simulink model "dc_servo_speed_estimation"  (R2020b)
settings: Solver=ode5  StartTime=0.0  StopTime=.25  FixedStep=.00001  RelTol=1e-6  AbsTol=1e-6
values from neighbouring files (symbols this model uses):
  encoder = 2000    [dc_servo_HighGainCommand_data.m]    (also in dc_servo_speed_estimation_data.m)
  f = 4e-4    (= 0.0004)    [dc_servo_HighGainCommand_data.m]    (also in dc_servo_speed_estimation_data.m)
  imax = 5    [dc_servo_HighGainCommand_data.m]    (also in dc_servo_speed_estimation_data.m)
  integrator_saturation = 10000    [dc_servo_HighGainCommand_data.m]    (also in dc_servo_speed_estimation_data.m)
  J = 6.0e-5    (= 6e-05)    [dc_servo_HighGainCommand_data.m]    (also in dc_servo_speed_estimation_data.m)
  KI = k*k    (= 10000)    [dc_servo_HighGainCommand_data.m]    (also in dc_servo_speed_estimation_data.m)
  Kp = k    (= 100)    [dc_servo_HighGainCommand_data.m]    (also in dc_servo_speed_estimation_data.m = 200)
  KT = 0.07    [dc_servo_HighGainCommand_data.m]    (also in dc_servo_speed_estimation_data.m)
  L = 0.002    [dc_servo_HighGainCommand_data.m]    (also in dc_servo_speed_estimation_data.m)
  l1 = p1 + p2 + p3 - f/J    (= 893.333333333)    [dc_servo_speed_estimation_data.m]
  l2 = p1*p2 + p1*p3 + p2*p3 -l1*(f/J)    (= 264044.444444)    [dc_servo_speed_estimation_data.m]
  l3 = -p1*p2*p3    (= -27000000)    [dc_servo_speed_estimation_data.m]
  load_torque = 0    [dc_servo_HighGainCommand_data.m]    (also in dc_servo_speed_estimation_data.m)
  omega0 = 0    [dc_servo_HighGainCommand_data.m]    (also in dc_servo_speed_estimation_data.m)
  R = 2    [dc_servo_HighGainCommand_data.m]    (also in dc_servo_speed_estimation_data.m)
  theta0 = 0    [dc_servo_HighGainCommand_data.m]    (also in dc_servo_speed_estimation_data.m)
  Ts = 0.001    [dc_servo_HighGainCommand_data.m]    (also in dc_servo_speed_estimation_data.m)
  vmax = 40    [dc_servo_HighGainCommand_data.m]    (also in dc_servo_speed_estimation_data.m)
libraries: simulink x1
settings Model: ExtModeTrigMode=oneshot  ExtModeArmWhenConnect=off  Creator=johnchiasson  LastModifiedBy=johnchiasson
settings DataIOCC: SaveFormat=Array  SignalLoggingSaveFormat=ModelDataLogs  SaveOutput=off  SaveTime=off  ReturnWorkspaceOutputs=off  SignalLoggingName=sigsOut
settings OptimizationCC: BlockReduction=off  BooleanDataType=off
settings DebuggingCC: SaveWithParameterizedLinksMsg=none  UnderspecifiedInitializationDetection=Classic  MergeDetectMultiDrivingBlocksExec=none  SignalResolutionControl=TryResolveAllWithWarning  MultiTaskDSMMsg=warning  MultiTaskCondExecSysMsg=none
settings HardwareCC: ProdBitPerPointer=32  ProdBitPerSizeT=32  ProdBitPerPtrDiffT=32  ProdLargestAtomicFloat=None  ProdIntDivRoundTo=Undefined  ProdEndianess=Unspecified  ProdWordSize=32  ProdHWDeviceType=32-bit Generic  TargetUnknown=on
settings ModelReferenceCC: PropagateSignalLabelsOutOfModel=off
settings GRTTargetCC: CombineOutputUpdateFcns=off  GRTInterface=on
settings ConfigComp: CovMetricSettings=dw  CovSaveCumulativeToWorkspaceVar=on  CovSaveSingleToWorkspaceVar=on

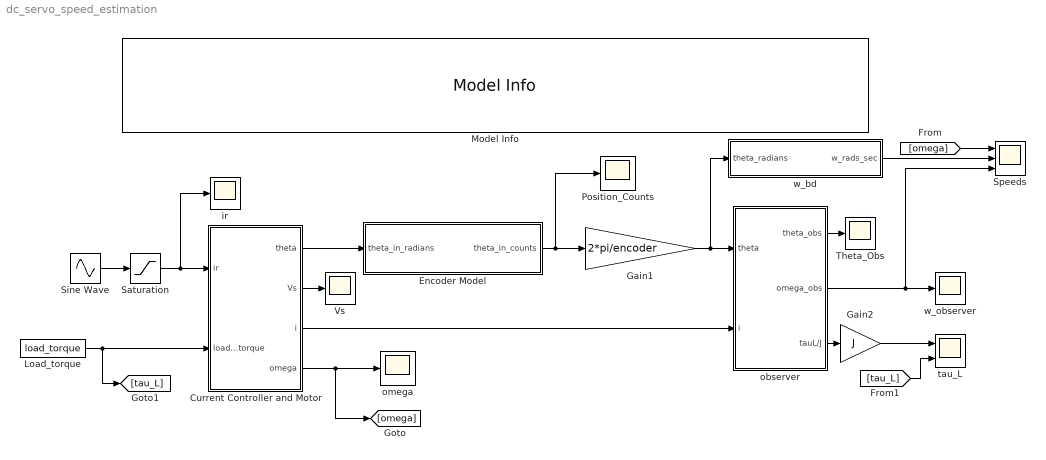
== system dc_servo_speed_estimation ==
  Current Controller and Motor : Subsystem
  Encoder Model : Subsystem
  Gain1 : Gain  Gain=2*pi/encoder  SaturateOnIntegerOverflow=on  OutDataTypeStr=Inherit: Same as input  ParamDataTypeStr=Inherit: Same as input
  Gain2 : Gain  Gain=J  SaturateOnIntegerOverflow=on  OutDataTypeStr=Inherit: Same as input  ParamDataTypeStr=Inherit: Same as input
  Load_torque : Constant  Value=load_torque
  Model Info : simulink/Model-Wide Utilities/Model Info  Frame=on  DisplayStringWithTags=|  HorizontalTextAlignment=Center  LeftAlignmentValue=0.5
      | Backward Difference Speed Estimator
      |  and 
      | Speed & Load Torque Estimator
  Position_Counts : Scope
  Saturation : Saturate  UpperLimit=imax  LowerLimit=-imax
  Sine Wave : Sin  Amplitude=0.5  Frequency=2*pi/0.2  SampleTime=0
  Speeds : Scope  NumInputPorts=3
  Theta_Obs : Scope
  Vs : Scope
  ir : Scope
  observer : Subsystem
  omega : Scope
  tau_L : Scope  NumInputPorts=2
  w_bd : Subsystem
  w_observer : Scope
  wires:
  Current Controller and Motor/4(omega) -> [omega], omega/1
  Load_torque/1 -> [tau_L], Current Controller and Motor/2(load_torque)
  Current Controller and Motor/2(Vs) -> Vs/1
  Current Controller and Motor/1(theta) -> Encoder Model/1(theta_in_radians)
  Saturation/1 -> Current Controller and Motor/1(ir), ir/1
  Gain1/1 -> w_bd/1(theta_radians), observer/1(theta)
  Encoder Model/1(theta_in_counts) -> Gain1/1, Position_Counts/1
  observer/1(theta_obs) -> Theta_Obs/1
  Current Controller and Motor/3(i) -> observer/2(i)
  observer/2(omega_obs) -> Speeds/3, w_observer/1
  w_bd/1(w_rads_sec) -> Speeds/2
  Sine Wave/1 -> Saturation/1
  observer/3(tauL/J) -> Gain2/1
  Gain2/1 -> tau_L/1
  [omega] -> Speeds/1
  [tau_L] -> tau_L/2

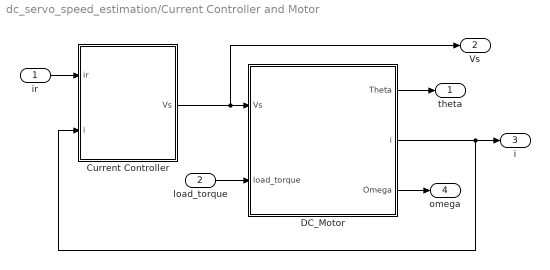
== system dc_servo_speed_estimation/Current Controller and Motor ==
  ir : Inport
  load_torque : Inport  Port=2
  Current Controller : Subsystem
  DC_Motor : Subsystem
  theta : Outport
  Vs : Outport  Port=2
  i : Outport  Port=3
  omega : Outport  Port=4
  wires:
  Current Controller/1(Vs) -> DC_Motor/1(Vs), Vs/1
  ir/1 -> Current Controller/1(ir)
  DC_Motor/3(Omega) -> omega/1
  DC_Motor/1(Theta) -> theta/1
  DC_Motor/2(i) -> i/1, Current Controller/2(i)
  load_torque/1 -> DC_Motor/2(load_torque)

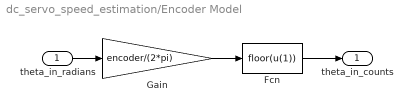
== system dc_servo_speed_estimation/Encoder Model ==
  theta_in_radians : Inport
  Fcn : Fcn  Expr=floor(u(1))
  Gain : Gain  Gain=encoder/(2*pi)  SaturateOnIntegerOverflow=on  OutDataTypeStr=Inherit: Same as input  ParamDataTypeStr=Inherit: Same as input
  theta_in_counts : Outport
  wires:
  Gain/1 -> Fcn/1
  theta_in_radians/1 -> Gain/1
  Fcn/1 -> theta_in_counts/1

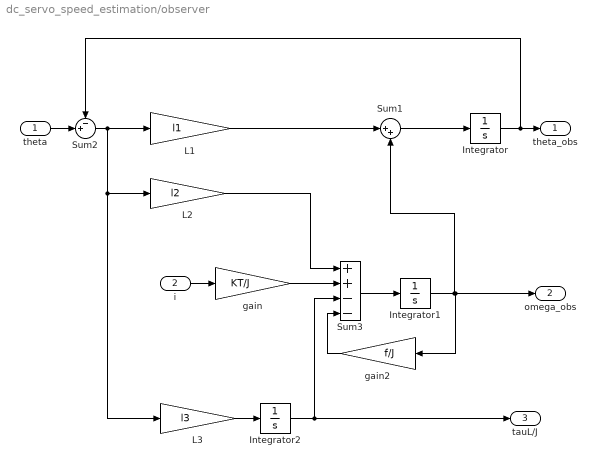
== system dc_servo_speed_estimation/observer ==
  theta : Inport
  i : Inport  Port=2
  Integrator : Integrator
  Integrator1 : Integrator
  Integrator2 : Integrator
  L1 : Gain  Gain=l1  SaturateOnIntegerOverflow=on  OutDataTypeStr=Inherit: Same as input  ParamDataTypeStr=Inherit: Same as input
  L2 : Gain  Gain=l2  SaturateOnIntegerOverflow=on  OutDataTypeStr=Inherit: Same as input  ParamDataTypeStr=Inherit: Same as input
  "L3 " : Gain  Gain=l3  SaturateOnIntegerOverflow=on  OutDataTypeStr=Inherit: Same as input  ParamDataTypeStr=Inherit: Same as input
  Sum1 : Sum  Inputs=|++  InputSameDT=on  SaturateOnIntegerOverflow=on  OutDataTypeStr=Inherit: Same as first input
  Sum2 : Sum  Inputs=-+|  InputSameDT=on  SaturateOnIntegerOverflow=on  OutDataTypeStr=Inherit: Same as first input
  Sum3 : Sum  Inputs=++--  InputSameDT=on  SaturateOnIntegerOverflow=on  OutDataTypeStr=Inherit: Same as first input
  gain : Gain  Gain=KT/J  SaturateOnIntegerOverflow=on  OutDataTypeStr=Inherit: Same as input  ParamDataTypeStr=Inherit: Same as input
  gain2 : Gain  Gain=f/J  SaturateOnIntegerOverflow=on  OutDataTypeStr=Inherit: Same as input  ParamDataTypeStr=Inherit: Same as input
  theta_obs : Outport
  omega_obs : Outport  Port=2
  tauL/J : Outport  Port=3
  wires:
  Sum2/1 -> L1/1, "L3 "/1, L2/1
  Sum3/1 -> Integrator1/1
  Integrator1/1 -> omega_obs/1, gain2/1, Sum1/2
  L1/1 -> Sum1/1
  Sum1/1 -> Integrator/1
  Integrator/1 -> Sum2/1, theta_obs/1
  theta/1 -> Sum2/2
  L2/1 -> Sum3/1
  gain/1 -> Sum3/2
  i/1 -> gain/1
  "L3 "/1 -> Integrator2/1
  Integrator2/1 -> Sum3/3, tauL/J/1
  gain2/1 -> Sum3/4

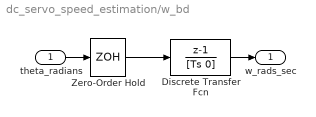
== system dc_servo_speed_estimation/w_bd ==
  theta_radians : Inport
  Discrete Transfer Fcn : DiscreteTransferFcn  Numerator=[1 -1]  Denominator=[Ts 0]  SampleTime=Ts
  Zero-Order Hold : ZeroOrderHold  SampleTime=Ts
  w_rads_sec : Outport
  wires:
  Discrete Transfer Fcn/1 -> w_rads_sec/1
  Zero-Order Hold/1 -> Discrete Transfer Fcn/1
  theta_radians/1 -> Zero-Order Hold/1

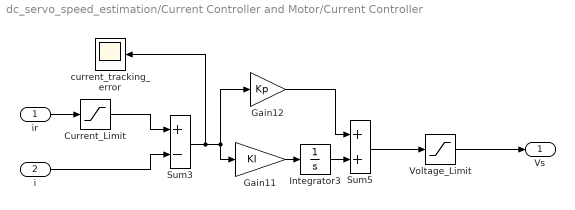
== system dc_servo_speed_estimation/Current Controller and Motor/Current Controller ==
  ir : Inport
  i : Inport  Port=2
  Current_Limit : Saturate  UpperLimit=imax  LowerLimit=-imax
  Gain11 : Gain  Gain=KI  SaturateOnIntegerOverflow=on  OutDataTypeStr=Inherit: Same as input  ParamDataTypeStr=Inherit: Same as input
  Gain12 : Gain  Gain=Kp  SaturateOnIntegerOverflow=on  OutDataTypeStr=Inherit: Same as input  ParamDataTypeStr=Inherit: Same as input
  Integrator3 : Integrator
  Sum3 : Sum  Inputs=+-  InputSameDT=on  SaturateOnIntegerOverflow=on  OutDataTypeStr=Inherit: Same as first input
  Sum5 : Sum  InputSameDT=on  SaturateOnIntegerOverflow=on  OutDataTypeStr=Inherit: Same as first input
  Voltage_Limit : Saturate  UpperLimit=vmax  LowerLimit=-vmax
  current_tracking_error : Scope
  Vs : Outport
  wires:
  Sum3/1 -> current_tracking_error/1, Gain11/1, Gain12/1
  Gain12/1 -> Sum5/1
  Integrator3/1 -> Sum5/2
  Gain11/1 -> Integrator3/1
  ir/1 -> Current_Limit/1
  Sum5/1 -> Voltage_Limit/1
  i/1 -> Sum3/2
  Voltage_Limit/1 -> Vs/1
  Current_Limit/1 -> Sum3/1

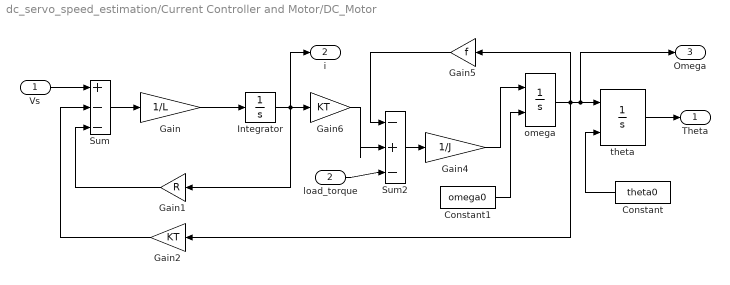
== system dc_servo_speed_estimation/Current Controller and Motor/DC_Motor ==
  Vs : Inport
  load_torque : Inport  Port=2
  Constant : Constant  Value=theta0
  Constant1 : Constant  Value=omega0
  Gain : Gain  Gain=1/L  SaturateOnIntegerOverflow=on  OutDataTypeStr=Inherit: Same as input  ParamDataTypeStr=Inherit: Same as input
  Gain1 : Gain  Gain=R  SaturateOnIntegerOverflow=on  OutDataTypeStr=Inherit: Same as input  ParamDataTypeStr=Inherit: Same as input
  Gain2 : Gain  Gain=KT  SaturateOnIntegerOverflow=on  OutDataTypeStr=Inherit: Same as input  ParamDataTypeStr=Inherit: Same as input
  Gain4 : Gain  Gain=1/J  SaturateOnIntegerOverflow=on  OutDataTypeStr=Inherit: Same as input  ParamDataTypeStr=Inherit: Same as input
  Gain5 : Gain  Gain=f  SaturateOnIntegerOverflow=on  OutDataTypeStr=Inherit: Same as input  ParamDataTypeStr=Inherit: Same as input
  Gain6 : Gain  Gain=KT  SaturateOnIntegerOverflow=on  OutDataTypeStr=Inherit: Same as input  ParamDataTypeStr=Inherit: Same as input
  Integrator : Integrator  LimitOutput=on  UpperSaturationLimit=integrator_saturation  LowerSaturationLimit=-integrator_saturation
  Sum : Sum  Inputs=+--  InputSameDT=on  SaturateOnIntegerOverflow=on  OutDataTypeStr=Inherit: Same as first input
  Sum2 : Sum  Inputs=|-+-  InputSameDT=on  SaturateOnIntegerOverflow=on  OutDataTypeStr=Inherit: Same as first input
  omega : Integrator  InitialConditionSource=external  LimitOutput=on  UpperSaturationLimit=integrator_saturation  LowerSaturationLimit=-integrator_saturation
  theta : Integrator  InitialConditionSource=external  LimitOutput=on  UpperSaturationLimit=integrator_saturation  LowerSaturationLimit=-integrator_saturation
  Theta : Outport
  i : Outport  Port=2
  Omega : Outport  Port=3
  wires:
  Gain/1 -> Integrator/1
  Gain1/1 -> Sum/3
  Sum/1 -> Gain/1
  Vs/1 -> Sum/1
  Integrator/1 -> Gain1/1, Gain6/1, i/1
  Sum2/1 -> Gain4/1
  Gain6/1 -> Sum2/2
  Gain4/1 -> omega/1
  load_torque/1 -> Sum2/3
  omega/1 -> Gain5/1, theta/1, Omega/1, Gain2/1
  Gain5/1 -> Sum2/1
  theta/1 -> Theta/1
  Gain2/1 -> Sum/2
  Constant/1 -> theta/2
  Constant1/1 -> omega/2
